simulink model "dc2dc_dcm"  (R2014a)
settings: Solver=ode45  StartTime=0.0  StopTime=10*Tmax  RelTol=1e-3
values from neighbouring files (symbols this model uses):
  a00c = sys(1).Ac(1,1)    [parameters.m]
  a00o = sys(1).Ao(1,1)    [parameters.m]
  a01c = sys(1).Ac(1,2)    [parameters.m]
  a01o = sys(1).Ao(1,2)    [parameters.m]
  a10c = sys(1).Ac(2,1)    [parameters.m]
  a10o = sys(1).Ao(2,1)    [parameters.m]
  a11c = sys(1).Ac(2,2)    [parameters.m]
  a11o = sys(1).Ao(2,2)    [parameters.m]
  b0c = sys(1).Bc(1)    [parameters.m]
  b0o = sys(1).Bo(1)    [parameters.m]
  b1c = sys(1).Bc(2)    [parameters.m]
  b1o = sys(1).Bo(2)    [parameters.m]
  D = cr*Vref/(cr*Vref + Vs)    (= 0.489795918367)    [parameters.m]
  i0 = 4.5    [parameters.m]
  T = 4e-6    (= 4e-06)    [parameters.m]
  v0 = 48    [parameters.m]
  Vref = 15    [parameters.m]    (also in parameters_dcmicrogrid.m = [48 48]; parameters_dcmicrogrid_hynger.m = [48 48])
  Vs = 20    [parameters.m]
  Vs_noise = 1    [parameters.m]
  Vtol = Vref / 200    (= 0.075)    [parameters.m]
settings Model: Creator=Luan Nguyen  LastModifiedBy=tjohnson
settings DataIOCC: SignalLoggingSaveFormat=ModelDataLogs
settings OptimizationCC: ExpressionDepthLimit=2147483647
settings DebuggingCC: UnderspecifiedInitializationDetection=Classic  MaxConsecutiveZCsMsg=none  MultiTaskDSMMsg=warning  MultiTaskCondExecSysMsg=none  StateNameClashWarn=warning
settings RTWCC: IncludeERTFirstTime=on

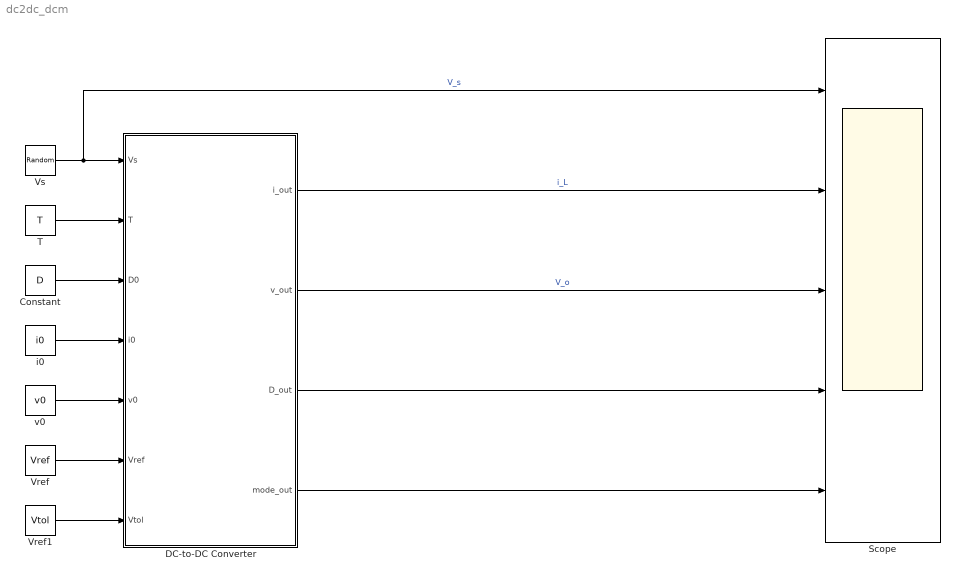
== system dc2dc_dcm ==
  Constant : Constant  Value=D
  DC-to-DC Converter : Stateflow chart  TreatAsAtomicUnit=on
  Scope : Scope  NumInputPorts=5
      settings: TimeRange=0.03  YMin=100~-4e-08~49.0151~0.6072~1  YMax=100~-5e-09~49.0151~0.6072~3  SaveName=dc2dc_ScopeData
  T : Constant  Value=T
  Vref : Constant  Value=Vref
  Vref1 : Constant  Value=Vtol
  Vs : RandomNumber  Mean=Vs  Variance=Vs_noise  SampleTime=T/10
  i0 : Constant  Value=i0
  v0 : Constant  Value=v0
  wires:
  DC-to-DC Converter/1(i_out) -> Scope/2  "i_L"
  DC-to-DC Converter/2(v_out) -> Scope/3  "V_o"
  T/1 -> DC-to-DC Converter/2(T)
  Vs/1 -> Scope/1, DC-to-DC Converter/1(Vs)  "V_s"
  i0/1 -> DC-to-DC Converter/4(i0)
  v0/1 -> DC-to-DC Converter/5(v0)
  Constant/1 -> DC-to-DC Converter/3(D0)
  Vref/1 -> DC-to-DC Converter/6(Vref)
  DC-to-DC Converter/3(D_out) -> Scope/4
  DC-to-DC Converter/4(mode_out) -> Scope/5
  Vref1/1 -> DC-to-DC Converter/7(Vtol)

== stateflow chart dc2dc_dcm/DC-to-DC Converter ==
  settings: updateMethod=CONTINUOUS
  state Discontinuous
    du:
    i_dot = a00d*i+a01d*v+b0d*Vs;
    v_dot = a10d*i+a11d*v+b1d*Vs;
    t_dot = 1;
    i_out =i;
    v_out = v;
    D_out=D;
    mode_out=3;
  state Charging
    du:
    i_dot = a00c*i+a01c*v+b0c*Vs;
    v_dot = a10c*i+a11c*v+b1c*Vs;
    t_dot = 1;
    i_out = i;
    v_out = v;
    D_out=D;
    mode_out=2;
  state Discharging
    du:
    i_dot = a00o*i+a01o*v+b0o*Vs;
    v_dot = a10o*i+a11o*v+b1o*Vs;
    t_dot = 1;
    i_out = i;
    v_out = v;
    D_out=D;
    mode_out=1;
  Discharging -> Discontinuous [order 1] : [i<=0&&0]
  Discontinuous -> Charging [order 1] : [v<=Vref-Vtol&&t>=T]
      | {t=0;}
  Discontinuous -> Discharging [order 2] : [v>=Vref+Vtol&&t>=T]
      | {t=0;}
  Charging -> Discharging : [v>=Vref+Vtol]
      | {t= 0;}
  Discharging -> Charging [order 2] : [v<=Vref-Vtol]
      | {t= 0;}
  (default) -> Discharging : {i = i0;
      | v = v0;
      | D=D0;}
  data: t local double; i_out output double; v_out output double; i local double; a00o local double; Vs input double =120; T input double; D0 input double; a01o local double; a10o local double; a11o local double; a00c local double; a01c local double; a10c local double; a11c local double; b0o local double; b1o local double; b0c local double; b1c local double; v local double; i0 input double; v0 input double; a01d local double; a10d local double; a11d local double; a00d local double; b0d local double; b1d local double; Vref input double =120; D local double; v1 local double; D_out output double; mode_out output double; Vtol input double =120
  data t settings: updateMethod=SF_CONTINUOUS_TIME_DATA
  data i settings: updateMethod=SF_CONTINUOUS_TIME_DATA
  data v settings: updateMethod=SF_CONTINUOUS_TIME_DATA
  data D settings: updateMethod=SF_CONTINUOUS_TIME_DATA
  data v1 settings: updateMethod=SF_CONTINUOUS_TIME_DATA
  data Vtol settings: description=Voltage tolerance (e.g., Vref / 100 is +/- 1% voltage ripple)
